simulink model "lab5simulink"  (R2020b)
settings: Solver=ode45  StartTime=0.0  StopTime=10  RelTol=1e-3
settings Model: Creator=wesle  LastModifiedBy=wesle
settings OptimizationCC: BooleanDataType=off

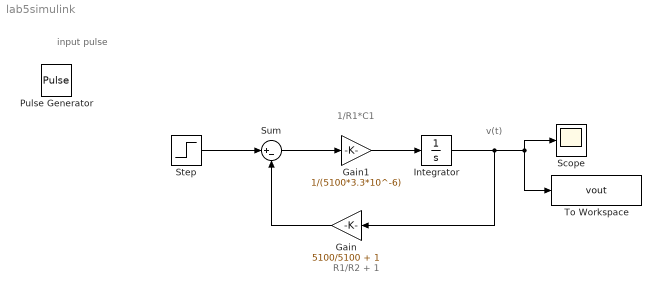
== system lab5simulink ==
  note: v(t)
  note: 1/R1*C1
  note: input pulse
  note: R1/R2 + 1
  Gain : Gain  Gain=5100/5100 + 1
  Gain1 : Gain  Gain=1/(5100*3.3*10^-6)
  Integrator : Integrator
  Pulse Generator : DiscretePulseGenerator  PulseType=Time based  Amplitude=60  Period=1000  PulseWidth=0.00016
  Scope : Scope
  Step : Step  After=2  SampleTime=0
  Sum : Sum  Inputs=|+-
  To Workspace : ToWorkspace  VariableName=vout  SampleTime=-1
  wires:
  Sum/1 -> Gain1/1
  Gain1/1 -> Integrator/1
  Gain/1 -> Sum/2
  Integrator/1 -> Gain/1, To Workspace/1, Scope/1
  Step/1 -> Sum/1
